simulink model "Sliding_Mode"  (R2020b)
settings: Solver=VariableStepAuto  StartTime=0.0  StopTime=15  RelTol=1e-3
settings Model: Creator=zhiyao  LastModifiedBy=zhiyao

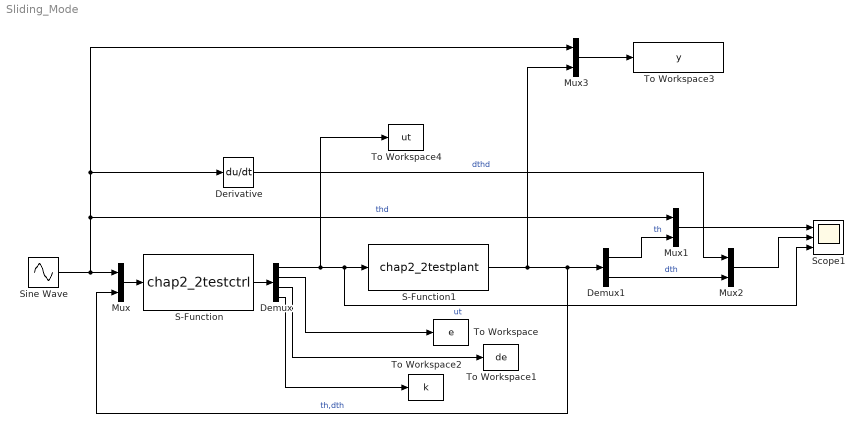
== system Sliding_Mode ==
  Demux : Demux
  Demux1 : Demux  Outputs=2
  Derivative : Derivative
  Mux{,1..3} (4 alike) : Mux  Inputs=2
  S-Function : S-Function  FunctionName=chap2_2testctrl  SFunctionDeploymentMode=off  EnableBusSupport=off
  S-Function1 : S-Function  FunctionName=chap2_2testplant  SFunctionDeploymentMode=off  EnableBusSupport=off
  Scope1 : Scope  NumInputPorts=3
  Sine Wave : Sin  SampleTime=0
  To Workspace : ToWorkspace  VariableName=e  SaveFormat=Timeseries  SampleTime=-1
  To Workspace1 : ToWorkspace  VariableName=de  SaveFormat=Timeseries  SampleTime=-1
  To Workspace2 : ToWorkspace  VariableName=k  SaveFormat=Timeseries  SampleTime=-1
  To Workspace3 : ToWorkspace  VariableName=y  SaveFormat=Timeseries  SampleTime=-1
  To Workspace4 : ToWorkspace  VariableName=ut  SaveFormat=Timeseries  SampleTime=-1
  wires:
  S-Function/1 -> Demux/1
  Demux/1 -> To Workspace4/1, Scope1/3, S-Function1/1  "ut"
  S-Function1/1 -> Mux3/2, Demux1/1, Mux/2  "th,dth"
  Mux/1 -> S-Function/1
  Sine Wave/1 -> Mux3/1, Derivative/1, Mux1/1, Mux/1  "thd"
  Demux/2 -> To Workspace/1
  Demux/3 -> To Workspace1/1
  Demux/4 -> To Workspace2/1
  Demux1/1 -> Mux1/2  "th"
  Demux1/2 -> Mux2/2  "dth"
  Derivative/1 -> Mux2/1  "dthd"
  Mux1/1 -> Scope1/1
  Mux2/1 -> Scope1/2
  Mux3/1 -> To Workspace3/1
